simulink model "ex3_new"  (R2013a)
settings: Solver=ode45  StartTime=0.0  StopTime=86400  RelTol=1e-3
settings Model: Creator=ahourai  LastModifiedBy=ahourai

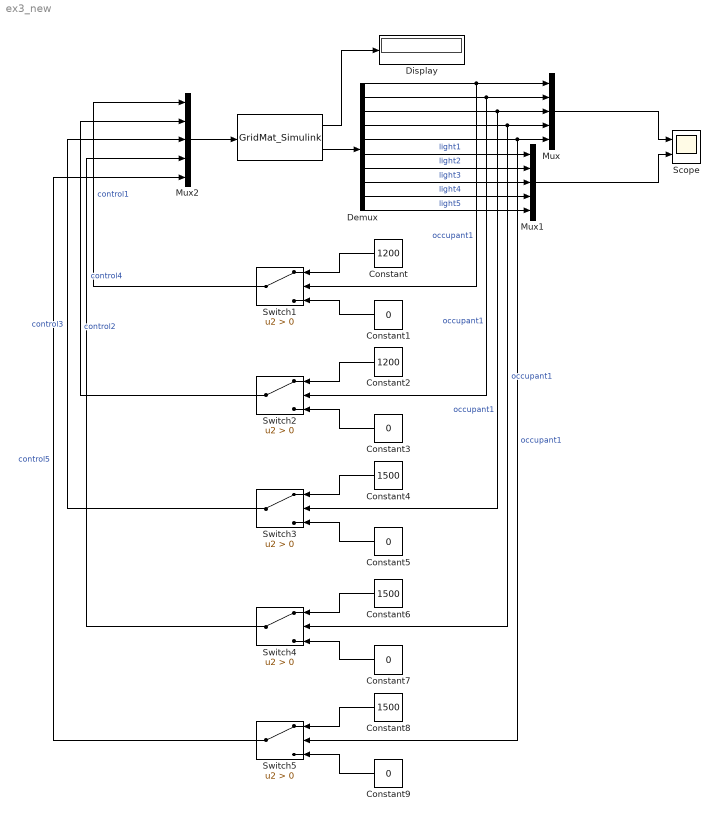
== system ex3_new ==
  " " : M-S-Function  FunctionName=GridMat_Simulink  Parameters=step,file,configuration  mask(GridMat Toolbox){step=60, file='mode', configuration='level_1'}
      mask prompts: step "Step Time"; file "GLM File"
      mask help: This bolck connects the Simulink part to GridLAB-D, and allow the design to model physical plant of grid Power.
      mask Display:
      | disp('GridLAB-D\n')
      | disp('\n (GridMat Toolbox) ');
  Constant : Constant  Value=1200
  Constant{1,3,5,7,9} (5 alike) : Constant  Value=0
  Constant2 : Constant  Value=1200
  Constant4 : Constant  Value=1500
  Constant6 : Constant  Value=1500
  Constant8 : Constant  Value=1500
  Demux : Demux  Outputs=10
  Display : Display
  Mux : Mux  Inputs=5
  Mux1 : Mux  Inputs=5
  Mux2 : Mux  Inputs=5
  Scope : Scope  NumInputPorts=2
      settings: YMin=0.2~1.2e+06  YMax=1~1.5e+06
  Switch{1..5} (5 alike) : Switch  Criteria=u2 > Threshold
  wires:
  " "/2 -> Demux/1
  Demux/1 -> Switch1/2, Mux/1  "occupant1"
  Demux/10 -> Mux1/5  "light5"
  Demux/9 -> Mux1/4  "light4"
  Demux/8 -> Mux1/3  "light3"
  Demux/7 -> Mux1/2  "light2"
  Demux/6 -> Mux1/1  "light1"
  Mux/1 -> Scope/1
  Mux1/1 -> Scope/2
  Mux2/1 -> " "/1
  Switch1/1 -> Mux2/1  "control1"
  Constant/1 -> Switch1/1
  Constant1/1 -> Switch1/3
  Demux/2 -> Switch2/2, Mux/2  "occupant1"
  Constant2/1 -> Switch2/1
  Constant3/1 -> Switch2/3
  Switch2/1 -> Mux2/2  "control2"
  Demux/3 -> Switch3/2, Mux/3  "occupant1"
  Constant4/1 -> Switch3/1
  Constant5/1 -> Switch3/3
  Switch3/1 -> Mux2/3  "control3"
  Demux/4 -> Switch4/2, Mux/4  "occupant1"
  Constant6/1 -> Switch4/1
  Constant7/1 -> Switch4/3
  Switch4/1 -> Mux2/4  "control4"
  Demux/5 -> Switch5/2, Mux/5  "occupant1"
  Constant8/1 -> Switch5/1
  Constant9/1 -> Switch5/3
  Switch5/1 -> Mux2/5  "control5"
  " "/1 -> Display/1
